simulink library "Pump_Main"  (Simulink 8.2)
settings: Solver=ode45  StartTime=0.0  StopTime=10.0  RelTol=1e-3
undefined symbols (not defined in the file): MassFlow, Temperature
libraries: carnot x3, simulink_extras x1
settings Model: Creator=lena.frank  LastModifiedBy=drhf

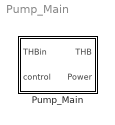
== system Pump_Main ==
  Pump_Main : Subsystem  mask(main pump){a0=2.7e4, a1=-1.2e4, a2=-3e-3, dia=0.025, t1=5, p0=3e5, IDchk=off, fluid_id=Water, mix=0, ua=1, mcp=500, tamb=20}
      mask prompts: a0 "constant coefficient a0 [Pa]"; a1 "linear coefficient a1 [Pa*s/kg]"; a2 "quadratic coefficient a2 [Pa*(s/kg)²]"; dia "diameter at in- and outlet [m]"; t1 "time constant in s"; p0 "system pressure in Pa"; IDchk "calculate static pressure in system"; fluid_id "fluid"; mix "percentage of fluid mix [0..1]"; ua "losses to ambient  in W/K"; mcp "thermal capacity in J/K"; tamb "ambient temperatature in °C"
      mask help:
      | This is the main pump in a circuit. Every circuit must have exactly ONE 'Pump_Main'. Use the 'pump_additional' blocks if you want to use more pumps.
      | Calculate massflow by solving the equations:
      |     pressure_drop = c + l*mdot + q*(mdot)²
      |     pump_pressure = a0 + a1*mdot +a2*(mdot)²
      |     with: pressure_drop = pump_pressure
      | The system pressure specified as parameter is the pressure at the outlet of the pump. All pressure drops in the circuit will reduce this pressure.
      mask init:
      | ID = IDchk*10000+10001;
      mask Help: web(fullfile(path_carnot('help'),'Pump_Main.html'),'-helpbrowser')
      mask TypeOptions fluid_id: Water | Air | Cotton Oil | Silicone Oil | Water-Glycol Mix | Tyfocor LS | Water (Constant 20°C) | Air (dry+ constant 20°C)
      mask Display:
      | plot(0,0,100,100,[40,70,40,30,30,40,60,70,70,60,40],[70,50,30,40,60,70,70,60,40,30,30])
      | port_label('input',1,'THB')
      | port_label('input',2,'ctr')
      | port_label('output',1,'THB')
      | port_label('output',2,'Pel')

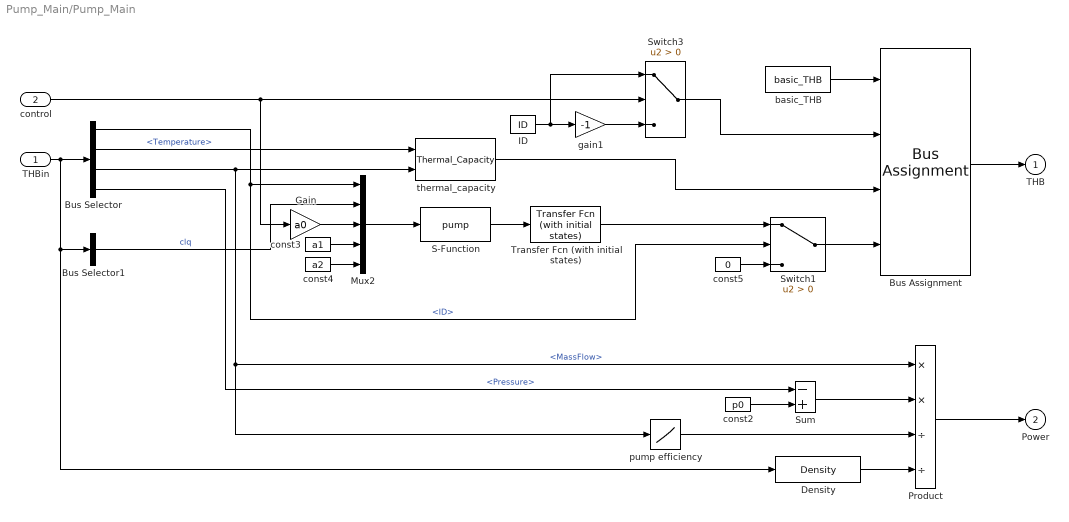
== system Pump_Main/Pump_Main ==
  THBin : Inport
  control : Inport  Port=2
  Bus Assignment : BusAssignment  AssignedSignals=ID,Temperature,MassFlow
  Bus Selector : BusSelector  OutputSignals=ID,Temperature,MassFlow,Pressure
  Bus Selector1 : BusSelector  OutputSignals=DPConstant,DPLinear,DPQuadratic  OutputAsBus=on
  Density : carnot/Basic/Material_Properties/Density  VariantControl=CarlibClassic  INPUTARGUMENTS=THB  DEBUGLEVEL=DEBUGLEVEL  MAXTOTALWARNINGS=inf  MAXCONSECUTIVEWARNINGS=inf  WRITETOFILE=0  FILENAME='errors.txt'
  Gain : Gain  Gain=a0
  ID : Constant  Value=ID
  Mux2 : Mux  Inputs=5
  Product : Product  Inputs=**//  SaturateOnIntegerOverflow=on  InputSameDT=on  OutDataTypeStr=Inherit: Same as first input
  S-Function : S-Function  FunctionName=pump  EnableBusSupport=off
  Sum : Sum  Inputs=-+
  Switch1 : Switch  Criteria=u2 > Threshold  SaturateOnIntegerOverflow=on  InputSameDT=on
  Switch3 : Switch  Criteria=u2 > Threshold  SaturateOnIntegerOverflow=on  InputSameDT=on
  Transfer Fcn (with initial states) : simulink_extras/Additional Linear/Transfer Fcn (with initial states)  N=[1]  D="[t1  1]"  X0=0
  basic_THB : carnot/Basic/Hydraulics/basic_THB  t=20  mdot=0  p=p0  ID=ID  fluid=fluid_id  mix=mix  dia=dia  hgt=0
  const2 : Constant  Value=p0
  const3 : Constant  Value=a1
  const4 : Constant  Value=a2
  const5 : Constant  Value=0
  gain1 : Gain  Gain=-1  SaturateOnIntegerOverflow=on  OutDataTypeStr=Inherit: Same as input  ParamDataTypeStr=Inherit: Same as input
  pump efficiency : Lookup  InputValues=0:1:5  Table=[0.001 0.5 0.7 0.7 0.5 0.001]  SaturateOnIntegerOverflow=on
  thermal_capacity : carnot/Basic/Thermal_Models/Thermal_Capacity  UA=ua  mcp=mcp  Tamb=tamb
  THB : Outport
  Power : Outport  Port=2
  wires:
  const2/1 -> Sum/2
  Sum/1 -> Product/2
  Product/1 -> Power/1
  Bus Selector/1 -> Mux2/1, Switch1/2  "<ID>"
  Bus Selector/4 -> Sum/1  "<Pressure>"
  Bus Selector/3 -> pump efficiency/1, Product/1, thermal_capacity/2  "<MassFlow>"
  Bus Selector/2 -> thermal_capacity/1  "<Temperature>"
  Mux2/1 -> S-Function/1
  pump efficiency/1 -> Product/3
  Density/1 -> Product/4
  S-Function/1 -> Transfer Fcn (with initial states)/1
  const3/1 -> Mux2/4
  const4/1 -> Mux2/5
  Gain/1 -> Mux2/3
  control/1 -> Gain/1, Switch3/2
  ID/1 -> gain1/1, Switch3/1
  gain1/1 -> Switch3/3
  Transfer Fcn (with initial states)/1 -> Switch1/1
  const5/1 -> Switch1/3
  basic_THB/1 -> Bus Assignment/1
  Bus Assignment/1 -> THB/1
  Switch3/1 -> Bus Assignment/2
  thermal_capacity/1 -> Bus Assignment/3
  Switch1/1 -> Bus Assignment/4
  THBin/1 -> Density/1, Bus Selector1/1, Bus Selector/1
  Bus Selector1/1 -> Mux2/2  "clq"
